simulink model "lab1"  (R2013a)
settings: Solver=ode5  StartTime=0.0  StopTime=inf  RelTol=1e-3
undefined symbols (not defined in the file or in its folder): National_Instruments, PCI
libraries: rtwinlib x2
settings Model: Creator=u_labelectro  LastModifiedBy=u_labelectro

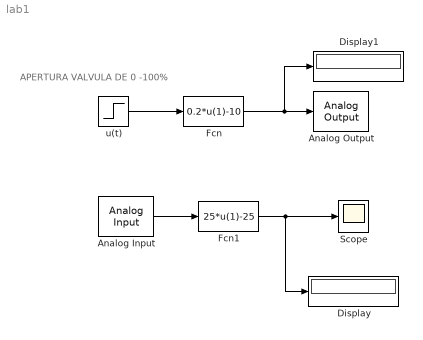
== system lab1 ==
  note: APERTURA VALVULA DE 0 -100%
  Analog Input : rtwinlib/Analog Input  SampleTime=0.1  MaxMissedTicks=10  ShowMissedTicks=off  YieldWhenWaiting=off  DrvName=National_Instruments/PCI-6229  DrvAddress=4294967295  DrvOptions=[0 0 0 0 0]  Channels=1  RangeMode=1  VoltRange=1  DataType=1
      settings: AttributesFormatString=National Instruments\nPCI-6229 [auto]
  Analog Output : rtwinlib/Analog Output  SampleTime=0.1  MaxMissedTicks=10  ShowMissedTicks=off  YieldWhenWaiting=off  DrvName=National_Instruments/PCI-6229  DrvAddress=4294967295  DrvOptions=[0 0 0 0 0]  Channels=1  RangeMode=1  VoltRange=1  InitialValue=[]  FinalValue=[]
      settings: AttributesFormatString=National Instruments\nPCI-6229 [auto]
  Display : Display
  Display1 : Display
  Fcn : Fcn  Expr=0.2*u(1)-10
  Fcn1 : Fcn  Expr=25*u(1)-25
  Scope : Scope
      settings: TimeRange=10
  u(t) : Step  Time=0  After=95  SampleTime=0
  wires:
  u(t)/1 -> Fcn/1
  Fcn/1 -> Display1/1, Analog Output/1
  Analog Input/1 -> Fcn1/1
  Fcn1/1 -> Display/1, Scope/1
